simulink model "QCar2_Virtual_Car2"  (R2023a)
settings: Solver=ode1  StartTime=0.0  StopTime=inf  FixedStep=cameraStepSize/10  RelTol=1e-3  EnableMultiTasking=on
PreLoadFcn:
  | QCarSetup
values from neighbouring files (symbols this model uses):
  cameraStepSize = 3e-2    (= 0.03)    [QCarSetup.m]
  path_x = [0.826 0.836 0.846 0.856 0.866 0.876 0.886 0.896 0.906 0.916 0.926 0.936 ... (740 elements, 740x1)]    [SDTS_Paths_6_2023.mat]
  path_x2 = [-0.614 -0.604 -0.594 -0.584 -0.574 -0.564 -0.554 -0.544 -0.534 -0.524 -0.514 -0.504 ... (1090 elements, 1090x1)]    [SDTS_Paths_6_2023.mat]
  path_x3 = [-0.614 -0.603821428571 -0.593642857143 -0.583464285714 -0.573285714286 -0.563107142857 -0.552928571429 -0.54275 -0.532571428571 -0.522392857143 -0.512214285714 -0.502035714286 ... (714 elements, 714x1)]    [SDTS_Paths_6_2023.mat]
  path_x4 = [-0.614 -0.604 -0.594 -0.584 -0.574 -0.564 -0.554 -0.544 -0.534 -0.524 -0.514 -0.504 ... (1761 elements, 1761x1)]    [SDTS_Paths_6_2023.mat]
  path_x5 = [1.436 1.42588571429 1.41577142857 1.40565714286 1.39554285714 1.38542857143 1.37531428571 1.3652 1.35508571429 1.34497142857 1.33485714286 1.32474285714 ... (574 elements, 574x1)]    [SDTS_Paths_6_2023.mat]
  path_x6 = [1.436 1.42588571429 1.41577142857 1.40565714286 1.39554285714 1.38542857143 1.37531428571 1.3652 1.35508571429 1.34497142857 1.33485714286 1.32474285714 ... (1288 elements, 1288x1)]    [SDTS_Paths_6_2023.mat]
  path_y = [-1.0887 -1.0887 -1.0887 -1.0887 -1.0887 -1.0887 -1.0887 -1.0887 -1.0887 -1.0887 -1.0887 -1.0887 ... (740 elements, 740x1)]    [SDTS_Paths_6_2023.mat]
  path_y2 = [-1.0887 -1.0887 -1.0887 -1.0887 -1.0887 -1.0887 -1.0887 -1.0887 -1.0887 -1.0887 -1.0887 -1.0887 ... (1090 elements, 1090x1)]    [SDTS_Paths_6_2023.mat]
  path_y3 = [-1.0887 -1.0887 -1.0887 -1.0887 -1.0887 -1.0887 -1.0887 -1.0887 -1.0887 -1.0887 -1.0887 -1.0887 ... (714 elements, 714x1)]    [SDTS_Paths_6_2023.mat]
  path_y4 = [-1.0887 -1.0887 -1.0887 -1.0887 -1.0887 -1.0887 -1.0887 -1.0887 -1.0887 -1.0887 -1.0887 -1.0887 ... (1761 elements, 1761x1)]    [SDTS_Paths_6_2023.mat]
  path_y5 = [-0.8157 -0.8157 -0.8157 -0.8157 -0.8157 -0.8157 -0.8157 -0.8157 -0.8157 -0.8157 -0.8157 -0.8157 ... (574 elements, 574x1)]    [SDTS_Paths_6_2023.mat]
  path_y6 = [-0.8157 -0.8157 -0.8157 -0.8157 -0.8157 -0.8157 -0.8157 -0.8157 -0.8157 -0.8157 -0.8157 -0.8157 ... (1288 elements, 1288x1)]    [SDTS_Paths_6_2023.mat]
undefined symbols (not defined in the file or in its folder): DiscIntNeverNeededParam, gcbh, height, Host, JPEG, left, qc_get_step_size, top, video_display_show, width
libraries: quarc_library x71, simulink_extras x12, simulink x5
(part 5 of 5)

== matlab function QCar2_Virtual_Car2/Randomizer/MATLAB Function ==
  data: Previous_Path input; Previous_Speed input; Path_Options input; Speed_Cmd_Base input; randomize input; Desired_Path output; Desired_Speed output; Accel_Limit output
function [Desired_Path, Desired_Speed,  Accel_Limit] = Random_Driving(Previous_Path, Previous_Speed, Path_Options, Speed_Cmd_Base, randomize)
%#codegen
Desired_Path = Previous_Path;
Desired_Speed = Previous_Speed;
Accel_Limit = 0;
num_Path_Options = sum (Path_Options);

if (randomize == 1) && (num_Path_Options > 0)
    random_Path = randi (num_Path_Options);
    valid_Paths = find (Path_Options);
    Desired_Path = valid_Paths (random_Path);
    Desired_Speed = Speed_Cmd_Base*randi(2);
    Accel_Limit = 0.1*randi(2);
end
if (Path_Options (Desired_Path) == 0)
    Desired_Path = Previous_Path;
end
end

== matlab function QCar2_Virtual_Car2/QCar/MATLAB Function ==
  data: previous_counter input; Camera_Select output; current_counter output
function [Camera_Select, current_counter] = Camera_Selection(previous_counter)
Camera_Select = [0 0 0 0 0 0];
current_counter = previous_counter + 1;
if current_counter == 11
    current_counter = 1;
end
if current_counter == 1
    Camera_Select = [0 0 0 0 1 0];
    % elseif current_counter == 2
    %     Camera_Select = [0 0 0 0 0 1];
    % elseif current_counter == 6
    %     Camera_Select = [0 0 0 0 1 0];
end

== matlab function QCar2_Virtual_Car2/Speed & Steering Commander/Traffic Zone 1/MATLAB Function2 ==
  data: Previous_State input; Speed_In input; Speed_Multi input; In_Zone input; Traffic_State output; Speed_Out output; Traffic_Light input
function [Traffic_State, Speed_Out]  = Traffic_Controller (Previous_State, Speed_In, Speed_Multi, In_Zone, Traffic_Light)
%#codegen
Traffic_State = Previous_State;
Speed_Out = Speed_In;

switch Traffic_State
    % Case 1 - Normal - either not in zone or green light, Case 2 - red
    % light and in zone
    
    case 1
        % Green light or not in zone
        Speed_Out = Speed_In;
        if (Traffic_Light == 0) && (In_Zone == 1)
            % Caught in the traffic controller's web!
            Traffic_State = 2;
        end
        
    case 2
        % Red light state
        Speed_Out = Speed_In * Speed_Multi;
        
        if (Traffic_Light == 1)
            % Green Light
            Traffic_State = 1;
        end
        
end
end

== matlab function QCar2_Virtual_Car2/Cameras/CSI Camera/Extract Center and Slope/Angle Check/MATLAB Function1 ==
  data: input input; output output; is_nan input; prev_output input
function output = fcn(input, is_nan, prev_output)
if is_nan == 1
    output = prev_output;
else
    output = input;
end

== matlab function QCar2_Virtual_Car2/Cameras/CSI Camera/Extract Center and Slope/MATLAB Function1 ==
  data: mean_x output; I input; mean_y output; angle output; m output; b output; score output
function [mean_x, mean_y, angle, m, b, score]  = Linear_Fit(I)
Size = size (I);
[rows, x] = find (I>0);
y = Size(1) - rows;
result = polyfit(y, x, 1);
m = result(1);
b = result(2);
angle=rad2deg (atan(m));
mean_y= mean (y);
mean_x=mean(x);
score = length(x);
end
